simulink model "A_Train_Sinario_Assi"  (R2019a)
settings: Solver=FixedStepDiscrete  StartTime=0.0  StopTime=50  FixedStep=1  RelTol=1e-3
libraries: simulink x1, powerlib_meascontrol x1
settings Model: Creator=hp  LastModifiedBy=Rahulw

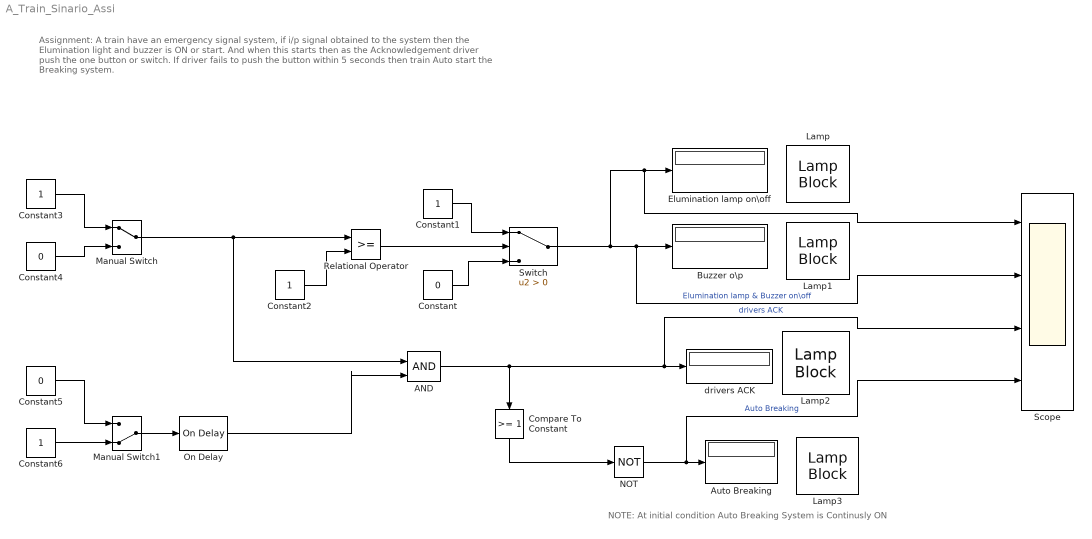
== system A_Train_Sinario_Assi ==
  note: NOTE: At initial condition Auto Breaking System is Continusly ON
  note: Assignment:
      | A train have an emergency signal system, if i/p signal obtained to the system then the Elumination light and buzzer is ON or start.
      | And when this starts then as the Acknowledgement driver push the one button or switch.
      | If driver fails to push the button within 5 seconds then train Auto start the Breaking system.
  AND : Logic  IconShape=distinctive  AllPortsSameDT=off  OutDataTypeStr=boolean
  Auto Breaking : Display
  Buzzer o\p : Display
  Compare To Constant : simulink/Logic and Bit Operations/Compare To Constant  relop=>=  const=1  OutDataTypeStr=boolean
  Constant : Constant  Value=0
  Constant{1..3,6} (4 alike) : Constant
  Constant4 : Constant  Value=0
  Constant5 : Constant  Value=0
  Elumination lamp on\off : Display
  Lamp{,1..3} (4 alike) : LampBlock  LabelPosition=Bottom
  Manual Switch : ManualSwitch
  Manual Switch1 : ManualSwitch  CurrentSetting=0
  NOT : Logic  Operator=NOT  IconShape=distinctive  AllPortsSameDT=off  OutDataTypeStr=boolean
  On Delay : powerlib_meascontrol/Logic/On Delay  DelayType=On delay  delay=5  ic=0  Ts=0
      settings: SourceProductName=Simscape Electrical
  Relational Operator : RelationalOperator  OutDataTypeStr=boolean  RndMeth=Simplest
  Scope : Scope  NumInputPorts=4
  Switch : Switch  Criteria=u2 > Threshold
  drivers ACK : Display
  wires:
  AND/1 -> Scope/3, drivers ACK/1, Compare To Constant/1  "drivers ACK"
  Constant/1 -> Switch/3
  Constant1/1 -> Switch/1
  Manual Switch/1 -> AND/1, Relational Operator/1
  Relational Operator/1 -> Switch/2
  Constant2/1 -> Relational Operator/2
  Switch/1 -> Scope/1, Elumination lamp on\off/1, Scope/2, Buzzer o\p/1  "Elumination lamp & Buzzer on\\off"
  On Delay/1 -> AND/2
  Constant3/1 -> Manual Switch/1
  Constant4/1 -> Manual Switch/2
  Constant6/1 -> Manual Switch1/2
  Constant5/1 -> Manual Switch1/1
  Manual Switch1/1 -> On Delay/1
  NOT/1 -> Scope/4, Auto Breaking/1  "Auto Breaking"
  Compare To Constant/1 -> NOT/1
